simulink model "Three_cell_Fuzzy_BMS"  (R2024b)
settings: Solver=VariableStepAuto  StartTime=0.0  StopTime=15  RelTol=1e-3
undefined symbols (not defined in the file): Ion, Lithium
libraries: spsSeriesRLCBranchLib x9, fuzblock x6, spsMeanLib x6, spsIdealSwitchLib x5, spsBatteryLib x3, spsDiodeLib x3, spsCurrentMeasurementLib x2, dspstat3 x2, spsDCVoltageSourceLib x1, spsGroundLib x1, spsPWMGenerator2LevelLib x1, sps_lib x1
settings Model: Creator=mridu  LastModifiedBy=Mridul
settings RTWCC: GPUComputeCapability=3.5

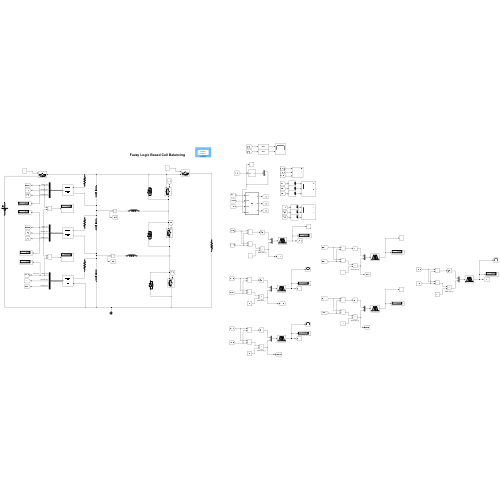
[thumbnail: Simulink's stored preview of the top-level diagram]
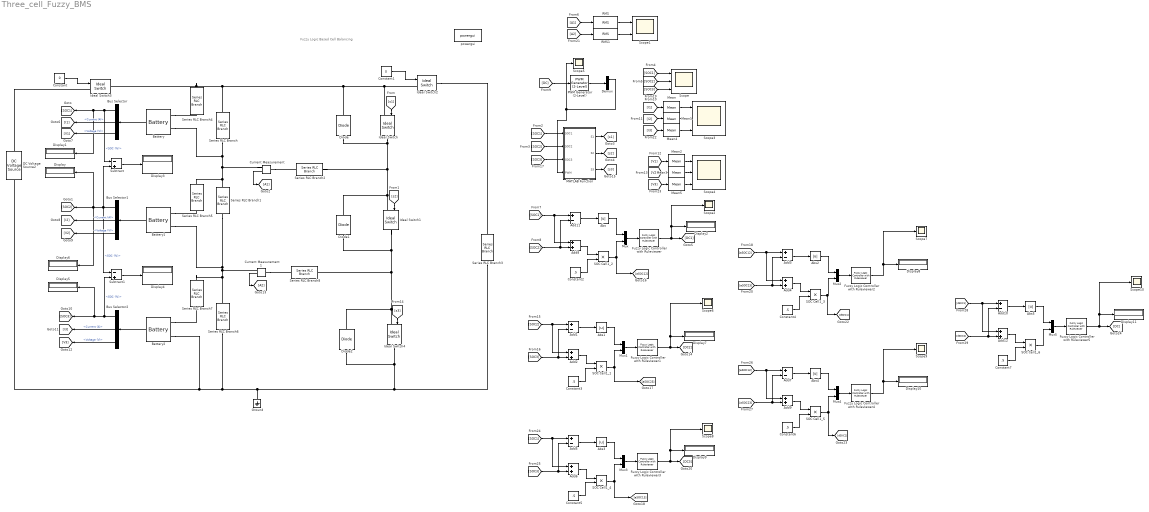
== system Three_cell_Fuzzy_BMS ==
  note: Fuzzy Logic Based Cell Balancing
  Abs{,1..5} (6 alike) : Abs  SaturateOnIntegerOverflow=off
  Add{1,3,5,7,10..11} (6 alike) : Sum  Inputs=+-
  Add{2,4,6,8..9,12} (6 alike) : Sum
  Battery : spsBatteryLib/Battery  BatType=Lithium-Ion  NomV=3.7  NomQ=3  SOC=70  Batt_Tr=0  PresetModel=on  MaxQ=3  MinV=2.775  FullV=4.3068  Dis_rate=1.3043  R=0.012333  Normal_OP=2.713  expZone="[3.9974     0.14739]"
  Battery1 : spsBatteryLib/Battery  BatType=Lithium-Ion  NomV=3.7  NomQ=3  SOC=74  Batt_Tr=0  PresetModel=on  MaxQ=3  MinV=2.775  FullV=4.3068  Dis_rate=1.3043  R=0.012333  Normal_OP=2.713  expZone="[3.9974     0.14739]"
  Battery2 : spsBatteryLib/Battery  BatType=Lithium-Ion  NomV=3.7  NomQ=3  SOC=76  Batt_Tr=0  PresetModel=on  MaxQ=3  MinV=2.775  FullV=4.3068  Dis_rate=1.3043  R=0.012333  Normal_OP=2.713  expZone="[3.9974     0.14739]"
  Bus Selector : BusSelector  OutputSignals=SOC (%),Current (A),Voltage (V)
  Bus Selector1 : BusSelector  OutputSignals=SOC (%),Current (A),Voltage (V)
  Bus Selector2 : BusSelector  OutputSignals=SOC (%),Current (A),Voltage (V)
  Constant : Constant  Value=0
  Constant1 : Constant  Value=0
  Constant{2..7} (6 alike) : Constant  Value=.5
  Current Measurement : spsCurrentMeasurementLib/Current Measurement  PhasorSimulation=off  OutputType=Complex  PSBequivalent=0
  Current Measurement1 : spsCurrentMeasurementLib/Current Measurement  PhasorSimulation=off  OutputType=Complex  PSBequivalent=0
  DC Voltage Source2 : spsDCVoltageSourceLib/DC Voltage Source  Amplitude=30  Measurements=None
  Demux : Demux  Outputs=2
  Diode : spsDiodeLib/Diode  Ron=0.001  Lon=0  Vf=0.8  IC=0  UseSnubber=0  Rs=500  Cs=250e-9  Measurements=off
  Diode1 : spsDiodeLib/Diode  Ron=0.001  Lon=0  Vf=0.8  IC=0  UseSnubber=0  Rs=500  Cs=250e-9  Measurements=off
  Diode2 : spsDiodeLib/Diode  Ron=0.001  Lon=0  Vf=0.8  IC=0  UseSnubber=0  Rs=500  Cs=250e-9  Measurements=off
  Display{,1..11} (12 alike) : Display
  Fuzzy Logic Controller with Ruleviewer : fuzblock/Fuzzy Logic  Controller  with Ruleviewer  fismatrix=Cell_Balance1  Ts=2
  Fuzzy Logic Controller with Ruleviewer1 : fuzblock/Fuzzy Logic  Controller  with Ruleviewer  fismatrix=Cell_Balance2  Ts=2
  Fuzzy Logic Controller with Ruleviewer2 : fuzblock/Fuzzy Logic  Controller  with Ruleviewer  fismatrix=Cell_Balance3  Ts=2
  Fuzzy Logic Controller with Ruleviewer3 : fuzblock/Fuzzy Logic  Controller  with Ruleviewer  fismatrix=Cell_Balance1  Ts=2
  Fuzzy Logic Controller with Ruleviewer4 : fuzblock/Fuzzy Logic  Controller  with Ruleviewer  fismatrix=Cell_Balance3  Ts=2
  Fuzzy Logic Controller with Ruleviewer5 : fuzblock/Fuzzy Logic  Controller  with Ruleviewer  fismatrix=Cell_Balance3  Ts=2
  Ground : spsGroundLib/Ground  LConnTagsString=a
  Ideal Switch{,1..4} (5 alike) : spsIdealSwitchLib/Ideal Switch  Ron=0.001  Lon=0  IC=0  Rs=1e5  Cs=inf  Measurements=off
  MATLAB Function : MATLAB Function  TreatAsAtomicUnit=on
  Mean{,1..5} (6 alike) : spsMeanLib/Mean  Freq=60  Vinit=0  Ts=0
  Mux{,1..5} (6 alike) : Mux  Inputs=2
  PWM Generator (2-Level) : spsPWMGenerator2LevelLib/PWM Generator (2-Level)  ModulatorType=Single-phase half-bridge (2 pulses)  ModulatorMode=Unsynchronized  Fc=500  Pc=0  nF=27  MinMax="[ -1  1 ]"  SamplingTechnique=Natural  ModulatingSignals=off  m=0.8  Freq=60  Phase=0  Ts=0  ShowCarrierOutport=off
  RMS : dspstat3/RMS  run=off  directionMode=Each column  dimension=1  InputProcessing=Columns as channels (frame based)  reset_popup=None
  RMS1 : dspstat3/RMS  run=off  directionMode=Each column  dimension=1  InputProcessing=Columns as channels (frame based)  reset_popup=None
  SOC Cell1_{1..6} (6 alike) : Product
  Scope : Scope  NumInputPorts=3
  Scope1 : Scope  NumInputPorts=2
  Scope{2,5..10} (7 alike) : Scope
  Scope3 : Scope  NumInputPorts=3
  Scope4 : Scope  NumInputPorts=3
  Series RLC Branch : spsSeriesRLCBranchLib/Series RLC Branch  LConnTagsString=__new0  RConnTagsString=__new0  BranchType=C  Resistance=1  Inductance=1e-3  SetiL0=off  InitialCurrent=0  Capacitance=1e-6  Setx0=off  InitialVoltage=0  Measurements=None
  Series RLC Branch1 : spsSeriesRLCBranchLib/Series RLC Branch  LConnTagsString=__new0  RConnTagsString=__new0  BranchType=C  Resistance=1  Inductance=1e-3  SetiL0=off  InitialCurrent=0  Capacitance=1e-6  Setx0=off  InitialVoltage=0  Measurements=None
  Series RLC Branch2 : spsSeriesRLCBranchLib/Series RLC Branch  LConnTagsString=__new0  RConnTagsString=__new0  BranchType=L  Resistance=1  Inductance=1e-3  SetiL0=off  InitialCurrent=0  Capacitance=1e-6  Setx0=off  InitialVoltage=0  Measurements=None
  Series RLC Branch3 : spsSeriesRLCBranchLib/Series RLC Branch  LConnTagsString=__new0  RConnTagsString=__new0  BranchType=R  Resistance=1  Inductance=1e-3  SetiL0=off  InitialCurrent=0  Capacitance=1e-6  Setx0=off  InitialVoltage=0  Measurements=None
  Series RLC Branch4 : spsSeriesRLCBranchLib/Series RLC Branch  LConnTagsString=__new0  RConnTagsString=__new0  BranchType=R  Resistance=0.01  Inductance=1e-3  SetiL0=off  InitialCurrent=0  Capacitance=1e-6  Setx0=off  InitialVoltage=0  Measurements=None
  Series RLC Branch5 : spsSeriesRLCBranchLib/Series RLC Branch  LConnTagsString=__new0  RConnTagsString=__new0  BranchType=R  Resistance=0.01  Inductance=1e-3  SetiL0=off  InitialCurrent=0  Capacitance=1e-6  Setx0=off  InitialVoltage=0  Measurements=None
  Series RLC Branch6 : spsSeriesRLCBranchLib/Series RLC Branch  LConnTagsString=__new0  RConnTagsString=__new0  BranchType=C  Resistance=1  Inductance=1e-3  SetiL0=off  InitialCurrent=0  Capacitance=1e-6  Setx0=off  InitialVoltage=0  Measurements=None
  Series RLC Branch7 : spsSeriesRLCBranchLib/Series RLC Branch  LConnTagsString=__new0  RConnTagsString=__new0  BranchType=R  Resistance=0.01  Inductance=1e-3  SetiL0=off  InitialCurrent=0  Capacitance=1e-6  Setx0=off  InitialVoltage=0  Measurements=None
  Series RLC Branch8 : spsSeriesRLCBranchLib/Series RLC Branch  LConnTagsString=__new0  RConnTagsString=__new0  BranchType=L  Resistance=1  Inductance=1e-3  SetiL0=off  InitialCurrent=0  Capacitance=1e-6  Setx0=off  InitialVoltage=0  Measurements=None
  Subtract : Sum  Inputs=-+
  Subtract1 : Sum  Inputs=-+
  powergui : sps_lib/powergui  Priority=1  SimulationMode=Discrete  SampleTime=.0001  frequency=60  Iterations=50  frequencyindice=0  Pbase=100e6  ErrMax=1e-4  UnitsV=kV  UnitsW=MW  buscounter=0  FunctionMessages=off  echomessages=off  EnableUseOfTLC=off  CurrentSourceSwitches=off  DisableSnubberDevices=off  DisableRonSwitches=off  DisableVfSwitches=off  DisplayEquations=off  AutomaticDiscreteSolvers=off  SolverType=Tustin/Backward Euler (TBE)  Interpol=off  ExternalGateDelay=off  methode=off  Ts=100  x0status=blocks  SPID=on  SwTol=0  HookPort=off  NonlinearTolerance=1e-4  nMaxIteration=100  ContinueOnMaxIteration=off  RestoreLinks=warning  ResistiveCurrentMeasurement=off  Frange=[0:2:500]  Ylog=off  Xlog=on  ShowGrid=off  save=off  variable=ZData  structure=0  ZoomFFT=off  StartTime=0.0  cycles=1  DisplayStyle=1  fundamental=60  FreqAxis=off  MaxFrequency=1000  frequencyindicesteady=1  RmsSteady=1  display=off
  wires:
  Battery/1 -> Bus Selector/1
  Battery1/1 -> Bus Selector1/1
  Constant/1 -> Ideal Switch3/1
  Constant1/1 -> Ideal Switch2/1
  Bus Selector1/1 -> Subtract1/1, Subtract/2, Display6/1, [SOC2], Display/1  "<SOC (%)>"
  Current Measurement/1 -> [A1]
  [s1] -> Ideal Switch/1
  [s2] -> Ideal Switch1/1
  MATLAB Function/2(S2) -> [s2]
  MATLAB Function/1(S1) -> [s1]
  [SOC1] -> MATLAB Function/1(SOC1)
  Demux/1 -> Scope5/1, MATLAB Function/4(PWM)
  [SOC2] -> MATLAB Function/2(SOC2)
  [DC] -> PWM Generator (2-Level)/1
  PWM Generator (2-Level)/1 -> Demux/1
  [SOC1] -> Scope/1
  [SOC2] -> Scope/2
  [A1] -> RMS/1
  RMS/1 -> Scope1/1
  [SOC1] -> Add8/1, Add11/1
  [SOC2] -> Add11/2, Add8/2
  Add8/1 -> SOC Cell1_2/1
  Constant2/1 -> SOC Cell1_2/2
  Add11/1 -> Abs/1
  Abs/1 -> Mux/1
  SOC Cell1_2/1 -> Mux/2, [aSOC12]
  Mux/1 -> Fuzzy Logic Controller with Ruleviewer/1
  Fuzzy Logic Controller with Ruleviewer/1 -> [DC1], Scope2/1, Display2/1
  Bus Selector/1 -> Subtract/1, [SOC1], Display1/1  "<SOC (%)>"
  Bus Selector/2 -> [I1]  "<Current (A)>"
  Bus Selector/3 -> [V1]  "<Voltage (V)>"
  Bus Selector1/2 -> [I2]  "<Current (A)>"
  Bus Selector1/3 -> [V2]  "<Voltage (V)>"
  Subtract/1 -> Display3/1
  [I1] -> Mean/1
  [I2] -> Mean1/1
  [V1] -> Mean2/1
  [V2] -> Mean3/1
  Mean/1 -> Scope3/1
  Mean1/1 -> Scope3/2
  Mean2/1 -> Scope4/1
  Mean3/1 -> Scope4/2
  Battery2/1 -> Bus Selector2/1
  Bus Selector2/3 -> [V3]  "<Voltage (V)>"
  Bus Selector2/2 -> [I3]  "<Current (A)>"
  Bus Selector2/1 -> Subtract1/2, Display5/1, [SOC3]  "<SOC (%)>"
  Current Measurement1/1 -> [A2]
  [s3] -> Ideal Switch4/1
  Subtract1/1 -> Display4/1
  Fuzzy Logic Controller with Ruleviewer1/1 -> Display7/1, Scope6/1, [DC2]
  Mux1/1 -> Fuzzy Logic Controller with Ruleviewer1/1
  SOC Cell1_1/1 -> [aSOC23], Mux1/2
  Abs1/1 -> Mux1/1
  Add1/1 -> Abs1/1
  Constant3/1 -> SOC Cell1_1/2
  Add2/1 -> SOC Cell1_1/1
  [SOC3] -> Add2/2, Add1/2
  [SOC2] -> Add1/1, Add2/1
  [SOC3] -> MATLAB Function/3(SOC3)
  MATLAB Function/3(S3) -> [s3]
  Fuzzy Logic Controller with Ruleviewer2/1 -> Display8/1, Scope7/1
  Mux2/1 -> Fuzzy Logic Controller with Ruleviewer2/1
  SOC Cell1_3/1 -> [dSOC1], Mux2/2
  Abs2/1 -> Mux2/1
  Add3/1 -> Abs2/1
  Constant4/1 -> SOC Cell1_3/2
  Add4/1 -> SOC Cell1_3/1
  [aSOC23] -> Add4/2, Add3/2
  [aSOC12] -> Add3/1, Add4/1
  [SOC3] -> Scope/3
  RMS1/1 -> Scope1/2
  [A2] -> RMS1/1
  Mean4/1 -> Scope3/3
  [I3] -> Mean4/1
  Mean5/1 -> Scope4/3
  [V3] -> Mean5/1
  Add5/1 -> Abs3/1
  Constant5/1 -> SOC Cell1_4/2
  SOC Cell1_4/1 -> Mux3/2, [aSOC13]
  Fuzzy Logic Controller with Ruleviewer3/1 -> [DC3], Scope8/1, Display9/1
  Abs3/1 -> Mux3/1
  Mux3/1 -> Fuzzy Logic Controller with Ruleviewer3/1
  [SOC3] -> Add5/2, Add6/2
  Add6/1 -> SOC Cell1_4/1
  [SOC1] -> Add6/1, Add5/1
  [aSOC13] -> Add9/1, Add7/1
  [aSOC23] -> Add7/2, Add9/2
  Add9/1 -> SOC Cell1_5/1
  Constant6/1 -> SOC Cell1_5/2
  Add7/1 -> Abs4/1
  Abs4/1 -> Mux4/1
  SOC Cell1_5/1 -> [dSOC2], Mux4/2
  Mux4/1 -> Fuzzy Logic Controller with Ruleviewer4/1
  Fuzzy Logic Controller with Ruleviewer4/1 -> Scope9/1, Display10/1
  [dSOC1] -> Add12/1, Add10/1
  [dSOC2] -> Add10/2, Add12/2
  Add12/1 -> SOC Cell1_6/1
  Constant7/1 -> SOC Cell1_6/2
  Add10/1 -> Abs5/1
  Abs5/1 -> Mux5/1
  SOC Cell1_6/1 -> Mux5/2
  Mux5/1 -> Fuzzy Logic Controller with Ruleviewer5/1
  Fuzzy Logic Controller with Ruleviewer5/1 -> [DC], Scope10/1, Display11/1
  connections:
  Ideal Switch2/LConn1 -- Ideal Switch/LConn1 -- Diode/RConn1 -- Series RLC Branch/LConn1 -- Series RLC Branch4/RConn1 -- Ideal Switch3/RConn1
  Ideal Switch3/LConn1 -- DC Voltage Source2/RConn1
  Diode2/RConn1 -- Diode1/LConn1 -- Ideal Switch1/RConn1 -- Series RLC Branch8/RConn1 -- Ideal Switch4/LConn1
  Ideal Switch2/RConn1 -- Series RLC Branch3/LConn1
  Series RLC Branch/RConn1 -- Current Measurement/RConn1 -- Series RLC Branch5/RConn1 -- Series RLC Branch1/LConn1 -- Battery/LConn2
  Ideal Switch/RConn1 -- Diode/LConn1 -- Series RLC Branch2/RConn1 -- Diode1/RConn1 -- Ideal Switch1/LConn1
  Current Measurement/LConn1 -- Series RLC Branch2/LConn1
  Battery/LConn1 -- Series RLC Branch4/LConn1
  Battery1/LConn1 -- Series RLC Branch5/LConn1
  Battery2/LConn1 -- Series RLC Branch7/LConn1
  Series RLC Branch7/RConn1 -- Battery1/LConn2 -- Series RLC Branch1/RConn1 -- Current Measurement1/RConn1 -- Series RLC Branch6/LConn1
  Current Measurement1/LConn1 -- Series RLC Branch8/LConn1
  Diode2/LConn1 -- Series RLC Branch3/RConn1 -- Ground/LConn1 -- Series RLC Branch6/RConn1 -- DC Voltage Source2/LConn1 -- Battery2/LConn2 -- Ideal Switch4/RConn1

== matlab function Three_cell_Fuzzy_BMS/MATLAB Function ==
  data: SOC1 input; S1 output; SOC2 input; SOC3 input; PWM input; S2 output; S3 output
function [S1, S2, S3] = fcn(SOC1, SOC2, SOC3, PWM)
    % Initialize the switching signals
    S1 = 0; S2 = 0; S3 = 0;

    % Find the cell with the highest and lowest SOC
    SOCs = [SOC1, SOC2, SOC3];
    [max_SOC, max_index] = max(SOCs); % Find maximum SOC and its index
    [min_SOC, min_index] = min(SOCs); % Find minimum SOC and its index

    % Logic for balancing the cells
    if max_index == 1 && min_index == 2
        % Cell 1 has the highest SOC, and Cell 2 has the lowest SOC
        S1 = PWM;  % Discharge Cell 1
        S2 = PWM;  % Charge Cell 2
        S3 = 0;    % Cell 3 remains idle
    elseif max_index == 1 && min_index == 3
        % Cell 1 has the highest SOC, and Cell 3 has the lowest SOC
        S1 = PWM;  % Discharge Cell 1
        S2 = 0;    % Cell 2 remains idle
        S3 = PWM;  % Charge Cell 3
    elseif max_index == 2 && min_index == 1
        % Cell 2 has the highest SOC, and Cell 1 has the lowest SOC
        S1 = PWM;  % Charge Cell 1
        S2 = PWM;  % Discharge Cell 2
        S3 = 0;    % Cell 3 remains idle
    elseif max_index == 2 && min_index == 3
        % Cell 2 has the highest SOC, and Cell 3 has the lowest SOC
        S1 = 0;    % Cell 1 remains idle
        S2 = PWM;  % Discharge Cell 2
        S3 = PWM;  % Charge Cell 3
    elseif max_index == 3 && min_index == 1
        % Cell 3 has the highest SOC, and Cell 1 has the lowest SOC
        S1 = PWM;  % Charge Cell 1
        S2 = 0;    % Cell 2 remains idle
        S3 = PWM;  % Discharge Cell 3
    elseif max_index == 3 && min_index == 2
        % Cell 3 has the highest SOC, and Cell 2 has the lowest SOC
        S1 = 0;    % Cell 1 remains idle
        S2 = PWM;  % Charge Cell 2
        S3 = PWM;  % Discharge Cell 3
    else
        % No balancing needed (all SOCs are equal or no significant difference)
        S1 = 0; S2 = 0; S3 = 0;
    end
end
